simulink model "statespace"  (R2024b)
settings: Solver=VariableStepAuto  StartTime=0.0  StopTime=10.0  RelTol=1e-3
model workspace (MAT data in the model file):
  Cyf = 60000
  Cyr = 60000
  Izz = 3000
  lf = 1.2
  lr = 1.5
  m = 1500
  vx0 = 20
settings Model: Creator=junhyeongdoh  LastModifiedBy=junhyeongdoh

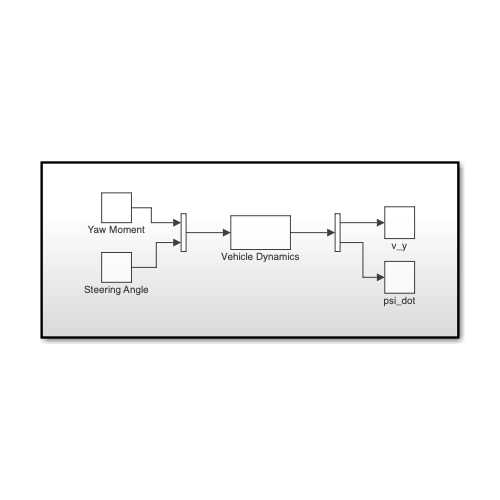
[thumbnail: Simulink's stored preview of the top-level diagram]
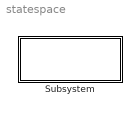
== system statespace ==
  Subsystem : Subsystem

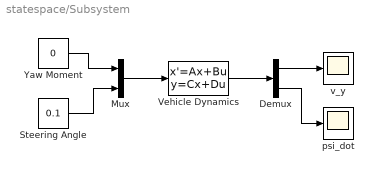
== system statespace/Subsystem ==
  Demux : Demux  Outputs=2
  Mux : Mux  Inputs=2
  Steering Angle : Constant  Value=0.1
  Vehicle Dynamics : StateSpace  A=[-(Cyf + Cyr)/(m*vx0),(-lf*Cyf + lr*Cyr)/(m*vx0) - vx0; (-lf*Cyf + lr*Cyr)/(Izz*vx0),-(lf^2*Cyf + lr^2*Cyr)/(Izz*vx0)]  B=[[Cyf/(m*vx0); lf*Cyf/Izz], [0; 1/(0.05*Izz)]]  C=[1 0; 0 1]  D=[0 0; 0 0]  InitialCondition=[0; 0]
  Yaw Moment : Constant  Value=0
  psi_dot : Scope
  v_y : Scope
  wires:
  Demux/1 -> v_y/1
  Mux/1 -> Vehicle Dynamics/1
  Yaw Moment/1 -> Mux/1
  Vehicle Dynamics/1 -> Demux/1
  Demux/2 -> psi_dot/1
  Steering Angle/1 -> Mux/2
